simulink model "lab06"  (Simulink 6.0)
settings: Solver=ode45  StartTime=0.0  StopTime=100  RelTol=1e-3
libraries: simulink x1
settings Model: LastModifiedBy=aluno

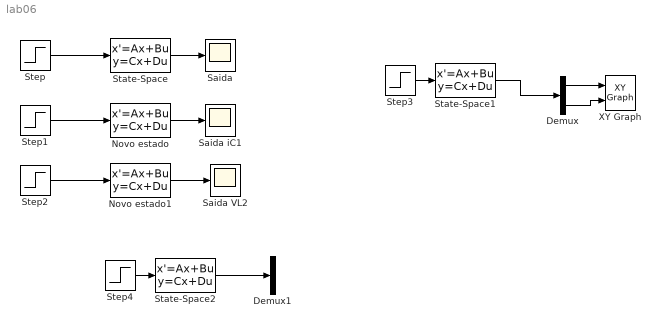
== system lab06 ==
  Demux : Demux  Outputs=2
  Demux1 : Demux  Outputs=2
  Novo estado : StateSpace  A="[-2 -2.828 0; 2.828 -2 0; 0  0 -4]"  B=[ 0; 3.366; -0.9427]  C="[0.4201    0.5941         0]"  D=0
  "Novo estado1 " : StateSpace  A="[-2 -2.828 0; 2.828 -2 0; 0  0 -4]"  B=[ 0; 3.366; -0.9427]  C="[-0.2802    0.792    2.828]"  D=0
  "Saida " : Scope
  Saida VL2 : Scope
      settings: SaveName=ScopeData2
  Saida iC1 : Scope
  State-Space : StateSpace  A=[-4 0 -2; 0 -4 1; 4 -4 0]  B=[2;0;0]  C=[0 1 0]  D=0
  State-Space1 : StateSpace  A=[-2 1; 1 -1]  B=[0; 0]  C=[1 0; 0 1]  D=[0; 0]  X0=[4; -5]
  State-Space2 : StateSpace  A=[-2 1; 1 -1]  B=[0; 0]  C=[1 0; 0 1]  D=[0; 0]  X0=[-5.257; -8.507]
  Step{,1..4} (5 alike) : Step  SampleTime=0
  XY Graph : simulink/Sinks/XY Graph  xmin=-5  xmax=5  ymin=-5  ymax=5  st=-1
  wires:
  Step/1 -> State-Space/1
  State-Space/1 -> "Saida "/1
  Step1/1 -> Novo estado/1
  Novo estado/1 -> Saida iC1/1
  Step2/1 -> "Novo estado1 "/1
  "Novo estado1 "/1 -> Saida VL2/1
  Step3/1 -> State-Space1/1
  State-Space2/1 -> Demux1/1
  Step4/1 -> State-Space2/1
  State-Space1/1 -> Demux/1
  Demux/1 -> XY Graph/1
  Demux/2 -> XY Graph/2
